simulink model "WormAndGearConstraint - Copy"  (R2024a)
settings: Solver=ode45  StartTime=0.0  StopTime=20  MaxStep=0.01  RelTol=1e-3
PreLoadFcn:
  | addpath(fullfile('WormAndGearConstraintSupport','Data'));
  | addpath(fullfile('WormAndGearConstraintSupport','Scripts'));
model workspace: external: MATLAB File WormAndGearConstraintParameters.m (data not in the file)
undefined symbols (not defined in the file or in its folder): Ion, Lithium, slewdrive, X, Y, Z
libraries: sm_lib x75, nesl_utility x40, neural x40, fl_lib x32, WormAndGearConstraintLibrary x24, spsSeriesRLCBranchLib x8, spsVoltageMeasurementLib x7, ee_lib x6, slpidlib x6, spsDiodeLib x5, spsBreakerLib x4, spsMosfetLib x3
(part 6 of 6)

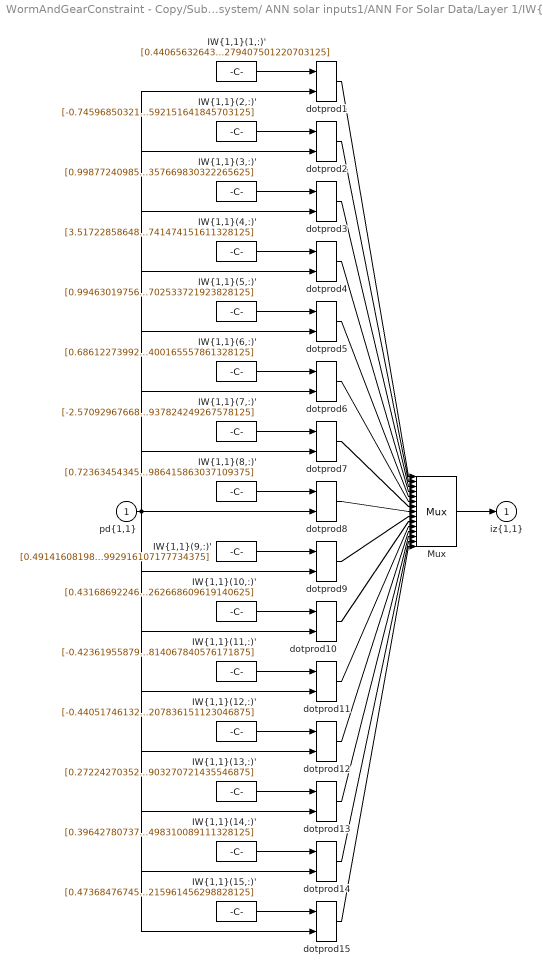
== system WormAndGearConstraint - Copy/Subsystem/ ANN solar inputs1/ANN For Solar Data/Layer 1/IW{1,1} ==
  "pd{1,1}" : Inport  PortDimensions=5
      mask Display: e = 0.06;c1 = [120 230 180]/255;c2 = ([120 230 180]+0)/(256+128);c3 = ([120 230 180]+128)/(256+128);patch([0 1 1 0],[0 0 1 1],c1);patch([0 1 1 1-e 1-e 0+e],[0 0 1 1-e 0+e 0+e],c2);patch([0 0 1 1-e 0+e 0+e],[0 1 1 1-e 1-e 0+e],c3);plot([0 1 1 0 0],[0 0 1 1 0]);
  "IW{1,1}(1,:)'" : Constant  Value=[0.440656326433005729459324584240675903856754302978515625;0.0082499057371298346874599616285195224918425083160400390625;-0.044099552646091534635619524351568543352186679840087890625;-0.00245166785449918260553214821584333549253642559051513671875;-1.5749584398746006019820242727291770279407501220703125]
      mask Display: e = 0.06;c1 = [120 150 230]/255;c2 = ([120 150 230]+0)/383;c3 = ([120 150 230]+128)/383;patch([0 1 1 0],[0 0 1 1],c1);patch([0 1 1 1-e 1-e 0+e],[0 0 1 1-e 0+e 0+e],c2);patch([0 0 1 1-e 0+e 0+e],[0 1 1 1-e 1-e 0+e],c3);plot([0 1 1 0 0],[0 0 1 1 0]);disp('Weights');
  "IW{1,1}(10,:)'" : Constant  Value=[0.43168692246912721000029478091164492070674896240234375;0.034341159783117192194623612522264011204242706298828125;-0.0175976984815091157254851594871070119552314281463623046875;0.00372555310842444774299675458451019949279725551605224609375;-2.406642111020334429127842668094672262668609619140625]
      mask Display: e = 0.06;c1 = [120 150 230]/255;c2 = ([120 150 230]+0)/383;c3 = ([120 150 230]+128)/383;patch([0 1 1 0],[0 0 1 1],c1);patch([0 1 1 1-e 1-e 0+e],[0 0 1 1-e 0+e 0+e],c2);patch([0 0 1 1-e 0+e 0+e],[0 1 1 1-e 1-e 0+e],c3);plot([0 1 1 0 0],[0 0 1 1 0]);disp('Weights');
  "IW{1,1}(11,:)'" : Constant  Value=[-0.42361955879776136413283893489278852939605712890625;1.10977633622082638709116508834995329380035400390625;-0.0835501550278960058992794301957474090158939361572265625;-2.61794715822211987443779435125179588794708251953125;-1.3518274325769723542833844476263038814067840576171875]
      mask Display: e = 0.06;c1 = [120 150 230]/255;c2 = ([120 150 230]+0)/383;c3 = ([120 150 230]+128)/383;patch([0 1 1 0],[0 0 1 1],c1);patch([0 1 1 1-e 1-e 0+e],[0 0 1 1-e 0+e 0+e],c2);patch([0 0 1 1-e 0+e 0+e],[0 1 1 1-e 1-e 0+e],c3);plot([0 1 1 0 0],[0 0 1 1 0]);disp('Weights');
  "IW{1,1}(12,:)'" : Constant  Value=[-0.440517461325625137025241429000743664801120758056640625;-0.01151117447380817053470547506321963737718760967254638671875;0.045248099003977693133293769278679974377155303955078125;0.0032734020863622557973027227262718952260911464691162109375;1.4633094238269730436030613418552093207836151123046875]
      mask Display: e = 0.06;c1 = [120 150 230]/255;c2 = ([120 150 230]+0)/383;c3 = ([120 150 230]+128)/383;patch([0 1 1 0],[0 0 1 1],c1);patch([0 1 1 1-e 1-e 0+e],[0 0 1 1-e 0+e 0+e],c2);patch([0 0 1 1-e 0+e 0+e],[0 1 1 1-e 1-e 0+e],c3);plot([0 1 1 0 0],[0 0 1 1 0]);disp('Weights');
  "IW{1,1}(13,:)'" : Constant  Value=[0.27224270352471890976886470525641925632953643798828125;-1.043836614745576429896800618735142052173614501953125;0.1896766694888755433456850596485310234129428863525390625;0.004672440805683443498796947324080974794924259185791015625;2.0409373300063844425267234328202903270721435546875]
      mask Display: e = 0.06;c1 = [120 150 230]/255;c2 = ([120 150 230]+0)/383;c3 = ([120 150 230]+128)/383;patch([0 1 1 0],[0 0 1 1],c1);patch([0 1 1 1-e 1-e 0+e],[0 0 1 1-e 0+e 0+e],c2);patch([0 0 1 1-e 0+e 0+e],[0 1 1 1-e 1-e 0+e],c3);plot([0 1 1 0 0],[0 0 1 1 0]);disp('Weights');
  "IW{1,1}(14,:)'" : Constant  Value=[0.396427807374588436761797538565588183701038360595703125;-1.789625106557950484642560695647262036800384521484375;-2.682230989124238629273122569429688155651092529296875;8.9025806104754980907500794273801147937774658203125;-4.12817824967732338592441010405309498310089111328125]
      mask Display: e = 0.06;c1 = [120 150 230]/255;c2 = ([120 150 230]+0)/383;c3 = ([120 150 230]+128)/383;patch([0 1 1 0],[0 0 1 1],c1);patch([0 1 1 1-e 1-e 0+e],[0 0 1 1-e 0+e 0+e],c2);patch([0 0 1 1-e 0+e 0+e],[0 1 1 1-e 1-e 0+e],c3);plot([0 1 1 0 0],[0 0 1 1 0]);disp('Weights');
  "IW{1,1}(15,:)'" : Constant  Value=[0.47368476745276277828367028632783330976963043212890625;-5.28165834570436576456131660961546003818511962890625;-0.581430249082355743439620709978044033050537109375;0.038405255237450079686123416422560694627463817596435546875;-2.768289678256326880045889993198215961456298828125]
      mask Display: e = 0.06;c1 = [120 150 230]/255;c2 = ([120 150 230]+0)/383;c3 = ([120 150 230]+128)/383;patch([0 1 1 0],[0 0 1 1],c1);patch([0 1 1 1-e 1-e 0+e],[0 0 1 1-e 0+e 0+e],c2);patch([0 0 1 1-e 0+e 0+e],[0 1 1 1-e 1-e 0+e],c3);plot([0 1 1 0 0],[0 0 1 1 0]);disp('Weights');
  "IW{1,1}(2,:)'" : Constant  Value=[-0.7459685032199796506091615810873918235301971435546875;0.03958991653606432070677811907444265671074390411376953125;-0.06880802029727785262824824030758463777601718902587890625;-0.00192728313709774300155341819618115550838410854339599609375;-3.09817162747569074809916855883784592151641845703125]
      mask Display: e = 0.06;c1 = [120 150 230]/255;c2 = ([120 150 230]+0)/383;c3 = ([120 150 230]+128)/383;patch([0 1 1 0],[0 0 1 1],c1);patch([0 1 1 1-e 1-e 0+e],[0 0 1 1-e 0+e 0+e],c2);patch([0 0 1 1-e 0+e 0+e],[0 1 1 1-e 1-e 0+e],c3);plot([0 1 1 0 0],[0 0 1 1 0]);disp('Weights');
  "IW{1,1}(3,:)'" : Constant  Value=[0.998772409858738274834877302055247128009796142578125;-0.119100118965819457006460879711084999144077301025390625;1.4734412523383586535175027165678329765796661376953125;0.1082246900612085227511016682910849340260028839111328125;-1.4500986091884959794384712949977256357669830322265625]
      mask Display: e = 0.06;c1 = [120 150 230]/255;c2 = ([120 150 230]+0)/383;c3 = ([120 150 230]+128)/383;patch([0 1 1 0],[0 0 1 1],c1);patch([0 1 1 1-e 1-e 0+e],[0 0 1 1-e 0+e 0+e],c2);patch([0 0 1 1-e 0+e 0+e],[0 1 1 1-e 1-e 0+e],c3);plot([0 1 1 0 0],[0 0 1 1 0]);disp('Weights');
  "IW{1,1}(4,:)'" : Constant  Value=[3.517228586487414876415869002812542021274566650390625;-11.1530312237673268072057908284477889537811279296875;-0.03467422529560158783734635790096945129334926605224609375;-0.0253280237128823415559963905252516269683837890625;1.7180664031691634807685886698891408741474151611328125]
      mask Display: e = 0.06;c1 = [120 150 230]/255;c2 = ([120 150 230]+0)/383;c3 = ([120 150 230]+128)/383;patch([0 1 1 0],[0 0 1 1],c1);patch([0 1 1 1-e 1-e 0+e],[0 0 1 1-e 0+e 0+e],c2);patch([0 0 1 1-e 0+e 0+e],[0 1 1 1-e 1-e 0+e],c3);plot([0 1 1 0 0],[0 0 1 1 0]);disp('Weights');
  "IW{1,1}(5,:)'" : Constant  Value=[0.9946301975619282753626748672104440629482269287109375;-0.1600082753687088743532740409136749804019927978515625;-1.521780916815078654735771124251186847686767578125;-0.1297648495221437048297019600795465521514415740966796875;-1.2414916778623013016158438404090702533721923828125]
      mask Display: e = 0.06;c1 = [120 150 230]/255;c2 = ([120 150 230]+0)/383;c3 = ([120 150 230]+128)/383;patch([0 1 1 0],[0 0 1 1],c1);patch([0 1 1 1-e 1-e 0+e],[0 0 1 1-e 0+e 0+e],c2);patch([0 0 1 1-e 0+e 0+e],[0 1 1 1-e 1-e 0+e],c3);plot([0 1 1 0 0],[0 0 1 1 0]);disp('Weights');
  "IW{1,1}(6,:)'" : Constant  Value=[0.68612273992241623599142030798248015344142913818359375;-0.104982209681928895239622079316177405416965484619140625;-0.613241164669414917653966767829842865467071533203125;-0.05920533907694876252225668622486409731209278106689453125;1.0022019309219019067569433900644071400165557861328125]
      mask Display: e = 0.06;c1 = [120 150 230]/255;c2 = ([120 150 230]+0)/383;c3 = ([120 150 230]+128)/383;patch([0 1 1 0],[0 0 1 1],c1);patch([0 1 1 1-e 1-e 0+e],[0 0 1 1-e 0+e 0+e],c2);patch([0 0 1 1-e 0+e 0+e],[0 1 1 1-e 1-e 0+e],c3);plot([0 1 1 0 0],[0 0 1 1 0]);disp('Weights');
  "IW{1,1}(7,:)'" : Constant  Value=[-2.57092967668512972778671610285528004169464111328125;-0.01478187733930325098441471709520556032657623291015625;-5.47678773959155140715893139713443815708160400390625;-0.6069798796372032345658453778014518320560455322265625;-1.7852945216614053425274732944671995937824249267578125]
      mask Display: e = 0.06;c1 = [120 150 230]/255;c2 = ([120 150 230]+0)/383;c3 = ([120 150 230]+128)/383;patch([0 1 1 0],[0 0 1 1],c1);patch([0 1 1 1-e 1-e 0+e],[0 0 1 1-e 0+e 0+e],c2);patch([0 0 1 1-e 0+e 0+e],[0 1 1 1-e 1-e 0+e],c3);plot([0 1 1 0 0],[0 0 1 1 0]);disp('Weights');
  "IW{1,1}(8,:)'" : Constant  Value=[0.72363454345364075503965750613133423030376434326171875;-0.162701561217215739940655794271151535212993621826171875;0.385534273778422253986519763202522881329059600830078125;0.0214664874822279548582937280798432766459882259368896484375;1.186058790761077119668698287568986415863037109375]
      mask Display: e = 0.06;c1 = [120 150 230]/255;c2 = ([120 150 230]+0)/383;c3 = ([120 150 230]+128)/383;patch([0 1 1 0],[0 0 1 1],c1);patch([0 1 1 1-e 1-e 0+e],[0 0 1 1-e 0+e 0+e],c2);patch([0 0 1 1-e 0+e 0+e],[0 1 1 1-e 1-e 0+e],c3);plot([0 1 1 0 0],[0 0 1 1 0]);disp('Weights');
  "IW{1,1}(9,:)'" : Constant  Value=[0.491416081983666319654702192565309815108776092529296875;-0.063370266488279758387847095946199260652065277099609375;-0.14774698755400617056210421651485376060009002685546875;-0.0228903924921436026373999794714109157212078571319580078125;0.65075914416514757387943745925440452992916107177734375]
      mask Display: e = 0.06;c1 = [120 150 230]/255;c2 = ([120 150 230]+0)/383;c3 = ([120 150 230]+128)/383;patch([0 1 1 0],[0 0 1 1],c1);patch([0 1 1 1-e 1-e 0+e],[0 0 1 1-e 0+e 0+e],c2);patch([0 0 1 1-e 0+e 0+e],[0 1 1 1-e 1-e 0+e],c3);plot([0 1 1 0 0],[0 0 1 1 0]);disp('Weights');
  Mux : Mux  Inputs=15
      mask Display: e = 0.06;c1 = [120 150 230]/255;c2 = ([120 150 230]+0)/383;c3 = ([120 150 230]+128)/383;patch([0 1 1 0],[0 0 1 1],c1);patch([0 1 1 1-e 1-e 0+e],[0 0 1 1-e 0+e 0+e],c2);patch([0 0 1 1-e 0+e 0+e],[0 1 1 1-e 1-e 0+e],c3);plot([0 1 1 0 0],[0 0 1 1 0]);disp('Mux');
  dotprod{1..15} (15 alike) : neural/Weight Functions/dotprod
  "iz{1,1}" : Outport
      mask Display: e = 0.06;c1 = [120 230 180]/255;c2 = ([120 230 180]+0)/(256+128);c3 = ([120 230 180]+128)/(256+128);patch([0 1 1 0],[0 0 1 1],c1);patch([0 1 1 1-e 1-e 0+e],[0 0 1 1-e 0+e 0+e],c2);patch([0 0 1 1-e 0+e 0+e],[0 1 1 1-e 1-e 0+e],c3);plot([0 1 1 0 0],[0 0 1 1 0]);
  wires:
  "IW{1,1}(1,:)'"/1 -> dotprod1/1
  "pd{1,1}"/1 -> dotprod1/2, dotprod2/2, dotprod3/2, dotprod4/2, dotprod5/2, dotprod6/2, dotprod7/2, dotprod8/2, dotprod9/2, dotprod10/2, dotprod11/2, dotprod12/2, dotprod13/2, dotprod14/2, dotprod15/2
  dotprod1/1 -> Mux/1
  "IW{1,1}(2,:)'"/1 -> dotprod2/1
  dotprod2/1 -> Mux/2
  "IW{1,1}(3,:)'"/1 -> dotprod3/1
  dotprod3/1 -> Mux/3
  "IW{1,1}(4,:)'"/1 -> dotprod4/1
  dotprod4/1 -> Mux/4
  "IW{1,1}(5,:)'"/1 -> dotprod5/1
  dotprod5/1 -> Mux/5
  "IW{1,1}(6,:)'"/1 -> dotprod6/1
  dotprod6/1 -> Mux/6
  "IW{1,1}(7,:)'"/1 -> dotprod7/1
  dotprod7/1 -> Mux/7
  "IW{1,1}(8,:)'"/1 -> dotprod8/1
  dotprod8/1 -> Mux/8
  "IW{1,1}(9,:)'"/1 -> dotprod9/1
  dotprod9/1 -> Mux/9
  "IW{1,1}(10,:)'"/1 -> dotprod10/1
  dotprod10/1 -> Mux/10
  "IW{1,1}(11,:)'"/1 -> dotprod11/1
  dotprod11/1 -> Mux/11
  "IW{1,1}(12,:)'"/1 -> dotprod12/1
  dotprod12/1 -> Mux/12
  "IW{1,1}(13,:)'"/1 -> dotprod13/1
  dotprod13/1 -> Mux/13
  "IW{1,1}(14,:)'"/1 -> dotprod14/1
  dotprod14/1 -> Mux/14
  "IW{1,1}(15,:)'"/1 -> dotprod15/1
  dotprod15/1 -> Mux/15
  Mux/1 -> "iz{1,1}"/1

== system WormAndGearConstraint - Copy/Subsystem/ ANN solar inputs1/ANN For Solar Data/Layer 2/Delays 1 ==
  "p{2}" : Inport  PortDimensions=15
      mask Display: e = 0.06;c1 = [120 230 180]/255;c2 = ([120 230 180]+0)/(256+128);c3 = ([120 230 180]+128)/(256+128);patch([0 1 1 0],[0 0 1 1],c1);patch([0 1 1 1-e 1-e 0+e],[0 0 1 1-e 0+e 0+e],c2);patch([0 0 1 1-e 0+e 0+e],[0 1 1 1-e 1-e 0+e],c3);plot([0 1 1 0 0],[0 0 1 1 0]);
  mux : Mux  Inputs=1
      mask Display: e = 0.06;c1 = [120 150 230]/255;c2 = ([120 150 230]+0)/383;c3 = ([120 150 230]+128)/383;patch([0 1 1 0],[0 0 1 1],c1);patch([0 1 1 1-e 1-e 0+e],[0 0 1 1-e 0+e 0+e],c2);patch([0 0 1 1-e 0+e 0+e],[0 1 1 1-e 1-e 0+e],c3);plot([0 1 1 0 0],[0 0 1 1 0]);disp('Mux')
  "pd{2,1}" : Outport
      mask Display: e = 0.06;c1 = [120 230 180]/255;c2 = ([120 230 180]+0)/(256+128);c3 = ([120 230 180]+128)/(256+128);patch([0 1 1 0],[0 0 1 1],c1);patch([0 1 1 1-e 1-e 0+e],[0 0 1 1-e 0+e 0+e],c2);patch([0 0 1 1-e 0+e 0+e],[0 1 1 1-e 1-e 0+e],c3);plot([0 1 1 0 0],[0 0 1 1 0]);
  wires:
  "p{2}"/1 -> mux/1
  mux/1 -> "pd{2,1}"/1

== system WormAndGearConstraint - Copy/Subsystem/ ANN solar inputs1/ANN For Solar Data/Layer 2/LW{2,1} ==
  "ad{2,1}" : Inport  PortDimensions=15
      mask Display: e = 0.06;c1 = [120 230 180]/255;c2 = ([120 230 180]+0)/(256+128);c3 = ([120 230 180]+128)/(256+128);patch([0 1 1 0],[0 0 1 1],c1);patch([0 1 1 1-e 1-e 0+e],[0 0 1 1-e 0+e 0+e],c2);patch([0 0 1 1-e 0+e 0+e],[0 1 1 1-e 1-e 0+e],c3);plot([0 1 1 0 0],[0 0 1 1 0]);
  "IW{2,1}(1,:)'" : Constant  Value=[-32.01745748567214633339972351677715778350830078125;1.31095166621215941660238968324847519397735595703125;0.42367758547066125540681014172150753438472747802734375;0.061422766084801093400269422772908001206815242767333984375;0.405265069982068959486554149407311342656612396240234375;2.479602125875937534971171771758235991001129150390625;0.07951932451130448720189036748706712387502193450927734375;2.0534231492268144592117096181027591228485107421875;-5.86111145507272457422232037060894072055816650390625;-2.668935957347304377407226638752035796642303466796875;0.0153001736286322957691918844602696481160819530487060546875;-33.27081827550976100837942794896662235260009765625;-0.361119480884813104371033887218800373375415802001953125;0.01235634921334839708695341187194571830332279205322265625;0.04399530117652304672670737772932625375688076019287109375]
      mask Display: e = 0.06;c1 = [120 150 230]/255;c2 = ([120 150 230]+0)/383;c3 = ([120 150 230]+128)/383;patch([0 1 1 0],[0 0 1 1],c1);patch([0 1 1 1-e 1-e 0+e],[0 0 1 1-e 0+e 0+e],c2);patch([0 0 1 1-e 0+e 0+e],[0 1 1 1-e 1-e 0+e],c3);plot([0 1 1 0 0],[0 0 1 1 0]);disp('weights');
  Mux : Mux  Inputs=1
      mask Display: e = 0.06;c1 = [120 150 230]/255;c2 = ([120 150 230]+0)/383;c3 = ([120 150 230]+128)/383;patch([0 1 1 0],[0 0 1 1],c1);patch([0 1 1 1-e 1-e 0+e],[0 0 1 1-e 0+e 0+e],c2);patch([0 0 1 1-e 0+e 0+e],[0 1 1 1-e 1-e 0+e],c3);plot([0 1 1 0 0],[0 0 1 1 0]);disp('Mux');
  dotprod1 : neural/Weight Functions/dotprod
  "lz{2,1}" : Outport
      mask Display: e = 0.06;c1 = [120 230 180]/255;c2 = ([120 230 180]+0)/(256+128);c3 = ([120 230 180]+128)/(256+128);patch([0 1 1 0],[0 0 1 1],c1);patch([0 1 1 1-e 1-e 0+e],[0 0 1 1-e 0+e 0+e],c2);patch([0 0 1 1-e 0+e 0+e],[0 1 1 1-e 1-e 0+e],c3);plot([0 1 1 0 0],[0 0 1 1 0]);
  wires:
  "IW{2,1}(1,:)'"/1 -> dotprod1/1
  "ad{2,1}"/1 -> dotprod1/2
  dotprod1/1 -> Mux/1
  Mux/1 -> "lz{2,1}"/1

== matlab function WormAndGearConstraint - Copy/Subsystem/ ANN solar inputs1/MATLAB Function1 ==
  data: lat input; output output; lon input
function output = generateInput(lat, lon)
    % Get the current date and time
    datetimeNow = datetime('now');
    [~, month, day , hour, ~, ~] = datevec(datetimeNow);

    % Create the output array
    output = [lat; lon; month; day; hour];
end

== matlab function WormAndGearConstraint - Copy/Subsystem/Subsystem1/battery bank /MATLAB Function ==
  data: SOC input; charge_ctrl output; discharge_ctrl output
function [charge_ctrl, discharge_ctrl] = battery_breaker_control(SOC)
% Inputs:
% SOC  - State of Charge (%)
% Outputs:
% charge_ctrl     - Control signal for the charger (1 = Allow charging, 0 = Stop charging)
% discharge_ctrl  - Control signal for the discharger (1 = Allow discharging, 0 = Stop discharging)

% Define SOC limits
SOC_max = 80; % Maximum SOC limit (%)
SOC_min = 20; % Minimum SOC limit (%)

% Default: Allow charging and discharging
charge_ctrl = 1;    % 1 = Charging allowed
discharge_ctrl = 1; % 1 = Discharging allowed

% Stop charging if SOC exceeds the maximum limit
if SOC > SOC_max
    charge_ctrl = 0; % Stop charging
end

% Stop discharging if SOC drops below the minimum limit
if SOC < SOC_min
    discharge_ctrl = 0; % Stop discharging
end
end

== matlab function WormAndGearConstraint - Copy/Subsystem/fresnal Algo for irradiance/MATLAB Function ==
  data: S2 input; Ir2 output; Incl input
function Ir2 = optics2(S2, Incl)
    
    %This function computes the reflection, absorption and transmission in
    %the glass to compute the irradiation to the PV cells, the heat absorbed 
    %in the glass and the radiation power absorbed in the PV cells,
    %it is based on Fresnel's laws, depending on the incident angle
    
    Ncell =  72;
    Acell =  0.0225;
    ng = 1.52;
    absg = 0.2;
    dg = 0.01;
    rpv = 0.15;
   

    % Fresnel equations 1st boundary
    r1p =  ( ng^2*cos(Incl) - sqrt(ng^2 - sin(Incl)^2) )^2/( ng^2*cos(Incl) + sqrt( ng^2 - sin(Incl)^2 ) )^2; %P polarization
    r1s =  ( cos(Incl) - sqrt(ng^2 - sin(Incl)^2) )^2/( cos(Incl) + sqrt( ng^2 - sin(Incl)^2 ) )^2; %S polarization
    r1 = 0.5*(r1p + r1s); %Effective reflectance
    t1 = 1-r1;

    nga = 1/ng; %refractive index glass -> air
    th2 = asin(sin(Incl)/ng);  %Snell's law to compute angle of incidence on 2nd boundary

    % Fresnel equations 2nd boundary
    r2p = ( nga^2*cos(th2) - sqrt(nga^2 - sin(th2)^2) )^2/( nga^2*cos(th2) + sqrt( nga^2 - sin(th2)^2 ) )^2 ;
    r2s = ( cos(th2) - sqrt(nga^2 - sin(th2)^2) )^2/( cos(th2) + sqrt( nga^2 - sin(th2)^2 ) )^2 ;
    r2 = 0.5*(r2p + r2s); %Effective reflectance
    t2 = 1 - r2;

    taug = exp(-absg*dg/cos(th2)); 
    
    %Total coefficients for infinite reflections between 2 parallel boundaries
    Transg = t1*taug*t2/(1 - r1*r2*taug^2);
    Reflg = r1 + (t1^2*taug^2*r2)/(1 - r1*r2*taug^2);
    Absg = 1 - Transg - Reflg; 

    Ir2 = S2*Transg; %Irradiation to the PV cells
    heatg = Acell*Ncell*Absg*S2; %heat absorbed in the glass
    powAbspv = Acell*Ncell*Transg*(1-rpv)*S2; %radiation power absorbed by PV cells. Part of it transforms in electrical power
    
end

== matlab function WormAndGearConstraint - Copy/Solar Array/MATLAB Function ==
  data: lat input; output output; lon input
function output = generateInput(lat, lon)
    % Get the current date and time
    datetimeNow = datetime('now');
    [~, month, day , hour, ~, ~] = datevec(datetimeNow);

    % Create the output array
    output = [lat; lon; month; day; hour];
end

== matlab function WormAndGearConstraint - Copy/MATLAB Function ==
  data: TimeVec input; SunAz output; Latitude input; Longitude input; UTCOffset input; SunEl output
function [SunAz, SunEl] = calculateSunPosition(TimeVec, Latitude, Longitude, UTCOffset)
    % Specify the output types and sizes explicitly to help Simulink understand
    % the expected dimensions of the outputs.
    coder.extrinsic('pvl_ephemeris'); % This tells Simulink that pvl_ephemeris is external.

    % Initialize outputs
    SunAz = 0; % Example value, replace with actual calculation
    SunEl = 0; % Example value, replace with actual calculation
    ApparentSunEl = 0; % Example value, replace with actual calculation
    SolarTime = 0; % Example value, replace with actual calculation

    % Extract time values from TimeVec input
    Year = TimeVec(1);
    Month = TimeVec(2);
    Day = TimeVec(3);
    Hour = TimeVec(4);
    Minute = TimeVec(5);
    Second = TimeVec(6);

    % Prepare the Time and Location structs
    TimeStruct = struct('year', Year, 'month', Month, 'day', Day, 'hour', Hour, ...
                        'minute', Minute, 'second', Second, 'UTCOffset', UTCOffset);

    LocationStruct = struct('latitude', Latitude, 'longitude', Longitude);

    % Call the pvl_ephemeris function to get sun position data
    [SunAz, SunEl] = pvl_ephemeris(TimeStruct, LocationStruct);
    
    % Alternatively, you can insert your own calculations for SunAz, SunEl, etc.
end

== stateflow chart WormAndGearConstraint - Copy/Solar Array/stateflow logic chart ==
  state Night_time
    during:
    pitch_upd = 0 ;
    yaw_upd = 0 ;
  state Cloudy
    entry:
    hold_pitch = pitch ;
    hold_yaw  = yaw ;
    during :
    pitch_upd = hold_pitch
    yaw_upd = hold_yaw;
    exit:
    pitch_upd = hold_pitch
    yaw_upd = hold_yaw;
  state Daytime
    during :
    pitch_upd = pitch;
    yaw_upd = yaw;
  Cloudy -> Night_time [order 2] : [abs(pitch) > 1.48353]
  Night_time -> Cloudy [order 1] : [ irradiance <450 && abs(pitch)<=1.48353 ]
  Night_time -> Daytime [order 2] : [abs(pitch)<=1.48353]
  Daytime -> Night_time [order 1] : [abs(pitch) > 1.48353]
  (default) -> Daytime
  Daytime -> Cloudy [order 2] : [ irradiance < 450 ]
  Cloudy -> Daytime [order 1] : [abs(pitch)<=1.48353 && irradiance>= 450]
  data: yaw input; yaw_upd output; pitch input; pitch_upd output; hold_yaw local double size=1; hold_pitch local double size=1; irradiance input

== matlab function WormAndGearConstraint - Copy/MATLAB Function1 ==
  data: unused input double size=1; timeVector output double size=[1 6]
function timeVector = extractTimeFromClock(~)
    datetimeNow = datetime('now');
    [year, month, day, hour, minute, second] = datevec(datetimeNow);
    timeVector = [year, month, day, hour, minute, second];
end

== matlab function WormAndGearConstraint - Copy/Subsystem/Battery Energy Storage System/MATLAB Function ==
  data: currentSoC input; newSoC output; chargeCurrent input; dischargeCurrent input; batteryCapacity input; timeStep input
function newSoC = SoCCalculation(currentSoC, chargeCurrent, dischargeCurrent, batteryCapacity, timeStep)
    % Calculate the new state of charge
    newSoC = currentSoC + (chargeCurrent - dischargeCurrent) * timeStep / (batteryCapacity * 3600); % Convert capacity to Wh
    % Limit the SoC between 0 and 1
    newSoC = max(0, min(0.90, newSoC));
end

== matlab function WormAndGearConstraint - Copy/Subsystem/Battery Energy Storage System/MATLAB Function1 ==
  data: PVPower input; chargeCurrent output; LoadDemand input; SoC input
function chargeCurrent = chargeControl(PVPower, LoadDemand, SoC)
    maxChargeCurrent = 50; % Maximum charging current in amps
    batteryVoltage = 12; % Example battery voltage
    if SoC < 0.95 % Charge battery if SoC is less than 95%
        excessPower = PVPower - LoadDemand;
        chargeCurrent = min(excessPower / batteryVoltage, maxChargeCurrent); % Adjust based on battery voltage
    else
        chargeCurrent = 0; % Stop charging if SoC >= 95%
    end
end

== matlab function WormAndGearConstraint - Copy/Subsystem/Battery Energy Storage System/MATLAB Function2 ==
  data: PVPower input; dischargeCurrent output; LoadDemand input; SoC input
function dischargeCurrent = dischargeControl(PVPower, LoadDemand, SoC)
    maxDischargeCurrent = 50; % Maximum discharging current in amps
    batteryVoltage = 12; % Example battery voltage
    if SoC > 0.2 % Discharge battery if SoC is more than 20%
        deficitPower = LoadDemand - PVPower;
        dischargeCurrent = min(deficitPower / batteryVoltage, maxDischargeCurrent); % Adjust based on battery voltage
    else
        dischargeCurrent = 0; % Stop discharging if SoC <= 20%
    end
end

== matlab function WormAndGearConstraint - Copy/Subsystem/Subsystem1/Battery Management system using fuzzy logic controller/MATLAB Function ==
  data: error input; outputQ1 output; outputQ2 output
function [outputQ1, outputQ2] = fuzzy_sugeno_bmss(error)
    % Define the membership function parameters for Error
    NE_params = [-100000 -100000 -50000 2500];  % trapmf for NE
    PE_params = [-2500 50000 100000 100000];    % trapmf for PE
    ZE_params = [0 0 0];                        % trimf for ZE
    
    % Evaluate membership functions for Error
    NE = trapmf(error, NE_params);  % Membership value for NE
    PE = trapmf(error, PE_params);  % Membership value for PE
    ZE = trimf(error, ZE_params);   % Membership value for ZE
    
    % Define rule outputs (constant values for Q1 and Q2)
    outputQ1_ON = 1;  % ON state for Q1
    outputQ1_OFF = 0; % OFF state for Q1
    
    outputQ2_ON = 1;  % ON state for Q2
    outputQ2_OFF = 0; % OFF state for Q2
    
    % Initialize outputs to NaN
    outputQ1 = NaN;
    outputQ2 = NaN;
    
    % Rule 1: If Error is NE, then Q1 is ON and Q2 is OFF
    if NE > 0
        outputQ1 = outputQ1_ON;
        outputQ2 = outputQ2_OFF;
    end
    
    % Rule 2: If Error is PE, then Q1 is ON and Q2 is OFF
    if PE > 0
        outputQ1 = outputQ1_ON;
        outputQ2 = outputQ2_OFF;
    end
    
    % Rule 3: If Error is ZE, then Q1 is OFF and Q2 is ON
    if ZE > 0
        outputQ1 = outputQ1_OFF;
        outputQ2 = outputQ2_ON;
    end
    
    % Defuzzification using weighted average method (wtaver)
    if (NE > 0) && (PE > 0)  % Overlap of NE and PE
        outputQ1 = (NE * outputQ1_ON + PE * outputQ1_ON) / (NE + PE);
        outputQ2 = (NE * outputQ2_OFF + PE * outputQ2_OFF) / (NE + PE);
    elseif (ZE > 0) && (NE > 0 || PE > 0)  % Overlap involving ZE
        outputQ1 = (ZE * outputQ1_OFF + NE * outputQ1_ON + PE * outputQ1_ON) / (ZE + NE + PE);
        outputQ2 = (ZE * outputQ2_ON + NE * outputQ2_OFF + PE * outputQ2_OFF) / (ZE + NE + PE);
    end
end
